simulink model "ThreePhaseVectorControl v2"  (R2020a)
settings: Solver=ode15s  StartTime=0.0  StopTime=2.5  MaxStep=1e-6  RelTol=1e-6
model workspace (MAT data in the model file):
  frequency = 1
values from neighbouring files (symbols this model uses):
  Buffer = 500    [PLLFYP.m]
  Ki_PLL = 0.005    [PLLFYP.m]
  Kp_PLL = 0.05    [PLLFYP.m]
  Kp_VSC = 500    [PLLFYP.m]
  Lf = 0.005    [PLLFYP.m]
  Lg = XR*Rg/(100*pi)    [PLLFYP.m]
  MPM_Ts = 1/5000    (= 0.0002)    [PLLFYP.m]
  Rf = 0.1    [PLLFYP.m]
  Rg = sqrt((1/(1+XR^2))*((500^2)/(Pn*SCR))^2)    [PLLFYP.m]
  Vdc = 2000    [PLLFYP.m]
  wL = 2*pi*50*Lf    (= 1.57079632679)    [PLLFYP.m]
  wn = 3000    [PLLFYP.m]
  zeta = 0.707    [PLLFYP.m]
undefined symbols (not defined in the file or in its folder): Ki_PQ, Kp_PQ, mpm_wc, plecs, Q, Q_KF, R, wb, wc, wc1, wc2
libraries: powerlib_meascontrol x57, powerlib x25, simulink x4, eeStairGenerator x4, powerlib_extras x2, cstblocks x2
(part 3 of 4)

== system ThreePhaseVectorControl v2/Vector Current Controller + PWM/KF_PLL/Kalman Filter-based PLL/Real Time Frequency Detection ==
  note: $x_{2_k}$
  note: $x_{1_k}$
  note: $\omega_k$
  r1 : Inport
  r2 : Inport  Port=2
  Trigger : TriggerPort  VariantControl=Variant  PortDimensions=1
  Add1 : Sum
  Discrete Derivative : simulink/Discrete/Discrete Derivative  gainval=1.0  ICPrevScaledInput=0.0  OutMin=[]  OutMax=[]  OutDataType=fixdt(1, 16)  OutScaling=2^-10  DoSatur=off
  Discrete Derivative1 : simulink/Discrete/Discrete Derivative  gainval=1.0  ICPrevScaledInput=0.0  OutMin=[]  OutMax=[]  OutDataType=fixdt(1, 16)  OutScaling=2^-10  DoSatur=off
  Divide4 : Product  Inputs=/*
  Product3 : Product
  Product4 : Product
  Square2 : Math  Operator=square  SaturateOnIntegerOverflow=on
  Square3 : Math  Operator=square  SaturateOnIntegerOverflow=on
  Subtract1 : Sum  Inputs=+-
  w_k : Outport
  wires:
  Subtract1/1 -> Divide4/2
  Product4/1 -> Subtract1/2
  r2/1 -> Square3/1, Discrete Derivative1/1, Product3/2
  Square3/1 -> Add1/2
  r1/1 -> Discrete Derivative/1, Product4/1, Square2/1
  Product3/1 -> Subtract1/1
  Square2/1 -> Add1/1
  Divide4/1 -> w_k/1
  Add1/1 -> Divide4/1
  Discrete Derivative1/1 -> Product4/2
  Discrete Derivative/1 -> Product3/1

== system ThreePhaseVectorControl v2/Vector Current Controller + PWM/KF_PLL/Kalman Filter-based PLL/abc-to-aphabetazero and Normalized ==
  note: $||v_{\alpha \beta k}^+||$
  note: $v_{\beta k}^+$
  note: $v_{\alpha k}^+$
  note: $r_{\beta_\omega}=cos(\theta_k^+)$
  note: $r_{\alpha__\omega}=sin(\theta_k^+)$
  note: $||v_{\alpha \beta k}^+||$
  Va S90 : Inport
  Vb S90 : Inport  Port=2
  Vc S90 : Inport  Port=3
  Trigger : TriggerPort  VariantControl=Variant  PortDimensions=1
  Add4 : Sum
  Demux : Demux  Outputs=3
  Divide : Product  Inputs=*/
  Divide2 : Product  Inputs=/*
  Mux : Mux  Inputs=3
  Square Root : Sqrt  SaturateOnIntegerOverflow=on
  Square6 : Math  Operator=square  SaturateOnIntegerOverflow=on
  Square7 : Math  Operator=square  SaturateOnIntegerOverflow=on
  Terminator : Terminator
  abc to Alpha-Beta-Zero : powerlib_meascontrol/Transformations/abc to Alpha-Beta-Zero
  r_bw : Outport
  r_aw : Outport  Port=2
  wires:
  abc to Alpha-Beta-Zero/1 -> Demux/1
  Square Root/1 -> Divide2/1, Divide/2
  Demux/2 -> Divide2/2, Square6/1
  Add4/1 -> Square Root/1
  Square7/1 -> Add4/1
  Square6/1 -> Add4/2
  Demux/1 -> Square7/1, Divide/1
  Demux/3 -> Terminator/1
  Mux/1 -> abc to Alpha-Beta-Zero/1
  Vc S90/1 -> Mux/3
  Divide2/1 -> r_bw/1
  Divide/1 -> r_aw/1
  Va S90/1 -> Mux/1
  Vb S90/1 -> Mux/2

== system ThreePhaseVectorControl v2/Vector Current Controller + PWM/KF_PLL/MPM (forcing Vq=0)/SRF-PLL for initialization ==
  VaB0 : Inport
  Add : Sum  Inputs=+-
  Add1 : Sum
  Alpha-Beta-Zero to dq0 : powerlib_meascontrol/Transformations/Alpha-Beta-Zero to dq0  Alignment=Aligned with phase A axis
  Constant : Constant  Value=2*pi
  Demux : Demux  Outputs=3
  Gain : Gain  Gain=Kp_PLL
  Integrator : Integrator  UpperSaturationLimit=2*pi  LowerSaturationLimit=0  IgnoreLimit=on
  Math Function : Math  Operator=mod  SignedPower=on  SaturateOnIntegerOverflow=on
  PI Controller : TransferFcn  Numerator=[1 Ki_PLL]  Denominator=[1 0]
  Terminator : Terminator
  Terminator1 : Terminator
  q reference : Step  Time=0  After=0  SampleTime=0
  w0 : Step  Time=0  After=2*pi*50  SampleTime=0
  SRF_theta : Outport
  wires:
  Demux/2 -> Add/1
  Math Function/1 -> SRF_theta/1, Alpha-Beta-Zero to dq0/2
  PI Controller/1 -> Add1/1
  q reference/1 -> Add/2
  Gain/1 -> PI Controller/1
  w0/1 -> Add1/2
  Demux/3 -> Terminator/1
  Add/1 -> Gain/1
  Alpha-Beta-Zero to dq0/1 -> Demux/1
  Constant/1 -> Math Function/2
  Integrator/1 -> Math Function/1
  Add1/1 -> Integrator/1
  VaB0/1 -> Alpha-Beta-Zero to dq0/1
  Demux/1 -> Terminator1/1

== system ThreePhaseVectorControl v2/Vector Current Controller + PWM/MPM/MPM (forcing Vq=0)/SRF-PLL for initialization ==
  VaB0 : Inport
  Add : Sum  Inputs=+-
  Add1 : Sum
  Alpha-Beta-Zero to dq0 : powerlib_meascontrol/Transformations/Alpha-Beta-Zero to dq0  Alignment=Aligned with phase A axis
  Constant : Constant  Value=2*pi
  Demux : Demux  Outputs=3
  Gain : Gain  Gain=Kp_PLL
  Integrator : Integrator  UpperSaturationLimit=2*pi  LowerSaturationLimit=0  IgnoreLimit=on
  Math Function : Math  Operator=mod  SignedPower=on  SaturateOnIntegerOverflow=on
  PI Controller : TransferFcn  Numerator=[1 Ki_PLL]  Denominator=[1 0]
  Terminator : Terminator
  Terminator1 : Terminator
  q reference : Step  Time=0  After=0  SampleTime=0
  w0 : Step  Time=0  After=2*pi*50  SampleTime=0
  SRF_theta : Outport
  wires:
  Demux/2 -> Add/1
  Math Function/1 -> SRF_theta/1, Alpha-Beta-Zero to dq0/2
  PI Controller/1 -> Add1/1
  q reference/1 -> Add/2
  Gain/1 -> PI Controller/1
  w0/1 -> Add1/2
  Demux/3 -> Terminator/1
  Add/1 -> Gain/1
  Alpha-Beta-Zero to dq0/1 -> Demux/1
  Constant/1 -> Math Function/2
  Integrator/1 -> Math Function/1
  Add1/1 -> Integrator/1
  VaB0/1 -> Alpha-Beta-Zero to dq0/1
  Demux/1 -> Terminator1/1

== system ThreePhaseVectorControl v2/Vector Current Controller + PWM/MPM/MPM (forcing Vq=0)/SRF-PLL for initialization1 ==
  VaB0 : Inport
  Add : Sum  Inputs=+-
  Add1 : Sum
  Alpha-Beta-Zero to dq0 : powerlib_meascontrol/Transformations/Alpha-Beta-Zero to dq0  Alignment=Aligned with phase A axis
  Constant : Constant  Value=2*pi
  Demux : Demux  Outputs=3
  Gain : Gain  Gain=Kp_PLL
  Integrator : Integrator  UpperSaturationLimit=2*pi  LowerSaturationLimit=0  IgnoreLimit=on
  Math Function : Math  Operator=mod  SignedPower=on  SaturateOnIntegerOverflow=on
  PI Controller : TransferFcn  Numerator=[1 Ki_PLL]  Denominator=[1 0]
  Terminator : Terminator
  Terminator1 : Terminator
  q reference : Step  Time=0  After=0  SampleTime=0
  w0 : Step  Time=0  After=2*pi*50  SampleTime=0
  SRF_theta : Outport
  wires:
  Demux/2 -> Add/1
  Math Function/1 -> SRF_theta/1, Alpha-Beta-Zero to dq0/2
  PI Controller/1 -> Add1/1
  q reference/1 -> Add/2
  Gain/1 -> PI Controller/1
  w0/1 -> Add1/2
  Demux/3 -> Terminator/1
  Add/1 -> Gain/1
  Alpha-Beta-Zero to dq0/1 -> Demux/1
  Constant/1 -> Math Function/2
  Integrator/1 -> Math Function/1
  Add1/1 -> Integrator/1
  VaB0/1 -> Alpha-Beta-Zero to dq0/1
  Demux/1 -> Terminator1/1

== system ThreePhaseVectorControl v2/Vector Current Controller + PWM/MPM/MPM (forcing Vq=0)/Vabc ==
  1 : Inport
  " InputMux " : Subsystem
      mask Display: disp('Mux')
  " S-Function " : S-Function  FunctionName=plecs  SFunctionDeploymentMode=off  EnableBusSupport=off
  wires:
  1/1 -> " InputMux "/1(In1)
  " InputMux "/1(Out) -> " S-Function "/1

== system ThreePhaseVectorControl v2/Vector Current Controller + PWM/MPM CF/MPM (forcing Vq=0)/SRF-PLL for initialization ==
  VaB0 : Inport
  Add : Sum  Inputs=+-
  Add1 : Sum
  Alpha-Beta-Zero to dq0 : powerlib_meascontrol/Transformations/Alpha-Beta-Zero to dq0  Alignment=Aligned with phase A axis
  Constant : Constant  Value=2*pi
  Demux : Demux  Outputs=3
  Gain : Gain  Gain=Kp_PLL
  Integrator : Integrator  UpperSaturationLimit=2*pi  LowerSaturationLimit=0  IgnoreLimit=on
  Math Function : Math  Operator=mod  SignedPower=on  SaturateOnIntegerOverflow=on
  PI Controller : TransferFcn  Numerator=[1 Ki_PLL]  Denominator=[1 0]
  Terminator : Terminator
  Terminator1 : Terminator
  q reference : Step  Time=0  After=0  SampleTime=0
  w0 : Step  Time=0  After=2*pi*50  SampleTime=0
  SRF_theta : Outport
  wires:
  Demux/2 -> Add/1
  Math Function/1 -> SRF_theta/1, Alpha-Beta-Zero to dq0/2
  PI Controller/1 -> Add1/1
  q reference/1 -> Add/2
  Gain/1 -> PI Controller/1
  w0/1 -> Add1/2
  Demux/3 -> Terminator/1
  Add/1 -> Gain/1
  Alpha-Beta-Zero to dq0/1 -> Demux/1
  Constant/1 -> Math Function/2
  Integrator/1 -> Math Function/1
  Add1/1 -> Integrator/1
  VaB0/1 -> Alpha-Beta-Zero to dq0/1
  Demux/1 -> Terminator1/1

== system ThreePhaseVectorControl v2/Vector Current Controller + PWM/MPM CF1/MPM (forcing Vq=0)/SRF-PLL for initialization ==
  VaB0 : Inport
  Add : Sum  Inputs=+-
  Add1 : Sum
  Alpha-Beta-Zero to dq0 : powerlib_meascontrol/Transformations/Alpha-Beta-Zero to dq0  Alignment=Aligned with phase A axis
  Constant : Constant  Value=2*pi
  Demux : Demux  Outputs=3
  Gain : Gain  Gain=Kp_PLL
  Integrator : Integrator  UpperSaturationLimit=2*pi  LowerSaturationLimit=0  IgnoreLimit=on
  Math Function : Math  Operator=mod  SignedPower=on  SaturateOnIntegerOverflow=on
  PI Controller : TransferFcn  Numerator=[1 Ki_PLL]  Denominator=[1 0]
  Terminator : Terminator
  Terminator1 : Terminator
  q reference : Step  Time=0  After=0  SampleTime=0
  w0 : Step  Time=0  After=2*pi*50  SampleTime=0
  SRF_theta : Outport
  wires:
  Demux/2 -> Add/1
  Math Function/1 -> SRF_theta/1, Alpha-Beta-Zero to dq0/2
  PI Controller/1 -> Add1/1
  q reference/1 -> Add/2
  Gain/1 -> PI Controller/1
  w0/1 -> Add1/2
  Demux/3 -> Terminator/1
  Add/1 -> Gain/1
  Alpha-Beta-Zero to dq0/1 -> Demux/1
  Constant/1 -> Math Function/2
  Integrator/1 -> Math Function/1
  Add1/1 -> Integrator/1
  VaB0/1 -> Alpha-Beta-Zero to dq0/1
  Demux/1 -> Terminator1/1

== system ThreePhaseVectorControl v2/Vector Current Controller + PWM/MPM//SRF CF/MPM (forcing Vq=0)/SRF-PLL for initialization ==
  VaB0 : Inport
  Add : Sum  Inputs=+-
  Add1 : Sum
  Alpha-Beta-Zero to dq0 : powerlib_meascontrol/Transformations/Alpha-Beta-Zero to dq0  Alignment=Aligned with phase A axis
  Constant : Constant  Value=2*pi
  Demux : Demux  Outputs=3
  Gain : Gain  Gain=Kp_PLL
  Integrator : Integrator  UpperSaturationLimit=2*pi  LowerSaturationLimit=0  IgnoreLimit=on
  Math Function : Math  Operator=mod  SignedPower=on  SaturateOnIntegerOverflow=on
  PI Controller : TransferFcn  Numerator=[1 Ki_PLL]  Denominator=[1 0]
  Terminator : Terminator
  Terminator1 : Terminator
  q reference : Step  Time=0  After=0  SampleTime=0
  w0 : Step  Time=0  After=2*pi*50  SampleTime=0
  SRF_theta : Outport
  wires:
  Demux/2 -> Add/1
  Math Function/1 -> SRF_theta/1, Alpha-Beta-Zero to dq0/2
  PI Controller/1 -> Add1/1
  q reference/1 -> Add/2
  Gain/1 -> PI Controller/1
  w0/1 -> Add1/2
  Demux/3 -> Terminator/1
  Add/1 -> Gain/1
  Alpha-Beta-Zero to dq0/1 -> Demux/1
  Constant/1 -> Math Function/2
  Integrator/1 -> Math Function/1
  Add1/1 -> Integrator/1
  VaB0/1 -> Alpha-Beta-Zero to dq0/1
  Demux/1 -> Terminator1/1

== system ThreePhaseVectorControl v2/Vector Current Controller + PWM/MPM//SRF CF/SRF_PLL/Vabc ==
  1 : Inport
  " InputMux " : Subsystem
      mask Display: disp('Mux')
  " S-Function " : S-Function  FunctionName=plecs  SFunctionDeploymentMode=off  EnableBusSupport=off
  wires:
  1/1 -> " InputMux "/1(In1)
  " InputMux "/1(Out) -> " S-Function "/1

== system ThreePhaseVectorControl v2/Vector Current Controller + PWM/MPM//SRF CF/SRF_PLL/Valphabeta ==
  1 : Inport
  " InputMux " : Subsystem
      mask Display: disp('Mux')
  " S-Function " : S-Function  FunctionName=plecs  SFunctionDeploymentMode=off  EnableBusSupport=off
  wires:
  1/1 -> " InputMux "/1(In1)
  " InputMux "/1(Out) -> " S-Function "/1

== system ThreePhaseVectorControl v2/Vector Current Controller + PWM/SRF_PLL/Vabc/ InputMux  ==
  In1 : Inport
  Convert1 : DataTypeConversion  SaturateOnIntegerOverflow=on  RndMeth=Zero
  Mux : Mux  Inputs=1
  Out : Outport
  wires:
  Convert1/1 -> Mux/1
  In1/1 -> Convert1/1
  Mux/1 -> Out/1

== system ThreePhaseVectorControl v2/Vector Current Controller + PWM/SRF_PLL/Valphabeta/ InputMux  ==
  In1 : Inport
  Convert1 : DataTypeConversion  SaturateOnIntegerOverflow=on  RndMeth=Zero
  Mux : Mux  Inputs=1
  Out : Outport
  wires:
  Convert1/1 -> Mux/1
  In1/1 -> Convert1/1
  Mux/1 -> Out/1

== system ThreePhaseVectorControl v2/Vector Current Controller + PWM/MPM/MPM (forcing Vq=0)/Vabc/ InputMux  ==
  In1 : Inport
  Convert1 : DataTypeConversion  SaturateOnIntegerOverflow=on  RndMeth=Zero
  Mux : Mux  Inputs=1
  Out : Outport
  wires:
  Convert1/1 -> Mux/1
  In1/1 -> Convert1/1
  Mux/1 -> Out/1

== system ThreePhaseVectorControl v2/Vector Current Controller + PWM/MPM//SRF CF/SRF_PLL/Vabc/ InputMux  ==
  In1 : Inport
  Convert1 : DataTypeConversion  SaturateOnIntegerOverflow=on  RndMeth=Zero
  Mux : Mux  Inputs=1
  Out : Outport
  wires:
  Convert1/1 -> Mux/1
  In1/1 -> Convert1/1
  Mux/1 -> Out/1

== system ThreePhaseVectorControl v2/Vector Current Controller + PWM/MPM//SRF CF/SRF_PLL/Valphabeta/ InputMux  ==
  In1 : Inport
  Convert1 : DataTypeConversion  SaturateOnIntegerOverflow=on  RndMeth=Zero
  Mux : Mux  Inputs=1
  Out : Outport
  wires:
  Convert1/1 -> Mux/1
  In1/1 -> Convert1/1
  Mux/1 -> Out/1

== matlab function ThreePhaseVectorControl v2/Vector Current Controller + PWM/MPM//SRF CF/MPM/MPM method 5 cycle ==
  data: x input; L input; timestep input; freq_guess input; outputfreq output
function outputfreq = Our_MPM_QR_pca(x,L,timestep,freq_guess)

%     Applies the Total Forward Backward Matrix Pencil Method to resolve the
%     synchrophasor of an input signal
%     Author: Lakshan Bernard, Sunny Goondram

% Inputs
% x:          one window of the timeseries
% L:          pencil parameter
% timestep:   time between sample points
% freq_guess: which phasors to report. NB: the method calculates all phasors
%             but the this just tells the algorithm to output phasor closest
%             to freq_guess
%             
% Outputs
% outputphasor:   a complex number representing the phasor relative to start
%                 of the window.
% outputfreq:     the frequency of the phasor. Note this is different to
%                 freq_guess
% eigS, residues: these contain all the frequency and phasor data

x = reshape(x, [], 1); %reshape data into column vector
N = length(x);
sampleoffset = (ceil(N/2)+1);
xold = x;

% Hyperparameters
DYNAMIC = 0;
if(DYNAMIC)
    epsilon=0.125;
    sys_order=floor((0.22/(50*timestep)));
else
    epsilon=0.05; %0.0050;
    sys_order=floor((N-sampleoffset)*1);
end

%% Filtering
    L1 = ceil(N/2);
    Y = hankel(x(1:N-L1), x(N-L1:N)); diagIdx = (N:-1:1)-L1;
    
    Y_mean = mean(Y,1);
    n = size(Y,1);
    matrix_mean = repmat(Y_mean,n,1); %creates a matrix with similar rows 
    centered_data = Y- matrix_mean;% centering the data by subtracting the mean
    M = ((centered_data')*centered_data)/(n-1);
    [V,D] = eig(M); %V are eigenvectors and D represents the eigenvalues 

    %sorting the eigen values in descending order
    lx = size(Y,2);
    eval = zeros(1,lx);
    eval = complex(eval, zeros(size(eval), class(eval)) );                      % Additional code added in
    for k = 1:lx
        eval(1,k) = D(k,k);
    end 
    [eval_sorted,I] = sort(eval,'descend');
    
    S = cumsum(abs(eval_sorted));
    limit = find((S/S(end))>0.9999999,1);
    if isempty(limit)                                                           % Additional code added in
        limit = 1;
    end
    limit = limit(1);
    evec_sorted = zeros(lx,limit);
    evec_sorted = complex(evec_sorted, zeros(size(evec_sorted), class(evec_sorted)) );    % Additional code added in
    for m =1:limit
        evec_sorted(:,m) = V(:,I(m));
    end
        
    %reconstruction
    princ_compon_limit = centered_data*evec_sorted;
    reconstructed = princ_compon_limit *(evec_sorted');
    reconstructed = reconstructed + matrix_mean;
    C = reconstructed;
 
    x1 = zeros(1,N);
    x1 = complex(x1, zeros(size(x1), class(x1)) );                              % Additional code added in
    for i=1:length(diagIdx) %averaging antidiagonals
        x1(i) = mean(diag(fliplr(C),diagIdx(i)));
    end    
    C = hankel(x1(1:N-L1), x1(N-L1:N)); 

    
%% Solving GEP

%perform the Column permutated QR decomposition for finding eigenvalues
%find the QR decomp for the all data matrix
[Q,R,E]=qr(C);

%rank estimation
order=0;

for i=1:length(diag(R))
    if abs(R(i,i))>=epsilon*abs(R(1,1))
        order=order+1;
    end
end

% Use permutation matrix to modify the Triangular R matrix
S=R*((E).');
% Create a new truncated pencil using the new matrix 
T1=S(1:order,1:L);
T2=S(1:order,2:L+1);
%modify the new pencil with diagonal of R matrix
Dinv=inv(diag(diag(R(1:order,1:order))));
T1dash=Dinv*T1;
T2dash=Dinv*T2;
%use the new pencil to find the eigenvalues
eigsS=eig(pinv(T2dash)*T1dash);
%remove the 0 eigenvalues;

eigsS(abs(eigsS)<10^-8)=[];
eigsS((abs(eigsS)<0.9)|(abs(eigsS)>1.1))=0;
order=length(eigsS);

%% Solving Complex Amplitudes
%form the linear system to solve for the complex amplitudes
ans_vec=xold(1+sampleoffset:sys_order+sampleoffset); %build answer vector (NB, this data hasnt been filtered :/)
coef_mat=zeros(sys_order,order);
coef_mat = complex(coef_mat, zeros(size(coef_mat), class(coef_mat)) );         % Additional code added in
for i=1:sys_order %build coefficient matrix
    for j=1:order
        coef_mat(i,j)=eigsS(j)^(i-1);
    end
end
residues=pinv(coef_mat)*ans_vec; %find the complex amplitudes


%% Estimating Frequency
freq = angle(eigsS)/(2*pi*timestep);
estfreq=freq_guess; %to report fundamental phasor replace with 50..
outputfreq = mean(freq( (freq>0.85*estfreq)&(freq<1.15*estfreq) ));

%% Reconstructing Phasor
%outputphasor = 2*sum(residues( (freq>0.85*freq_guess)&(freq<1.15*freq_guess) ));

== matlab function ThreePhaseVectorControl v2/Vector Current Controller + PWM/KF_PLL/KF//GAM/Kalman Filter/KF_Vb ==
  data: y_k input; v_fk output; R input; Q input; w_k input; V_fk_S90 output
function [v_fk, V_fk_S90] = fcn(y_k, R, Q, w_k)
 
persistent P_k;
persistent xhat_k;

% Initialize xhat and Phat
    if isempty(P_k)
        P_k = eye(2);
    end
    if isempty(xhat_k)
        xhat_k = zeros(2, 1);
    end
    
% Variables for KF
    Ts = 10e-6;       
    phi_k = [cos(w_k*Ts) sin(w_k*Ts); -sin(w_k*Ts) cos(w_k*Ts)];  
    F_k = [1 0];


K = phi_k * P_k * F_k' / (F_k * P_k * F_k' + R);        %K_gain * Phat_next * F_k' /(F_k*Phat_next*F_k' + R);    
xhat_k1 = phi_k * xhat_k + K * (y_k - F_k * xhat_k);
P_k1 = phi_k * P_k * phi_k' - K * F_k * P_k * phi_k' + Q;

xhat_k = xhat_k1;
P_k = P_k1;

% Output
v_fk = xhat_k1(1);
V_fk_S90 = xhat_k1(2);


 
end

== matlab function ThreePhaseVectorControl v2/Vector Current Controller + PWM/KF_PLL/KF//GAM/Kalman Filter/KF_Vc ==
  data: y_k input; v_fk output; R input; Q input; w_k input; V_fk_S90 output
function [v_fk, V_fk_S90] = fcn(y_k, R, Q, w_k)
 
persistent P_k;
persistent xhat_k;

% Initialize xhat and Phat
    if isempty(P_k)
        P_k = eye(2);
    end
    if isempty(xhat_k)
        xhat_k = zeros(2, 1);
    end

% Variables for KF
    Ts = 10e-6;       
    phi_k = [cos(w_k*Ts) sin(w_k*Ts); -sin(w_k*Ts) cos(w_k*Ts)];  %phi_k = [1 0; 0 1];
    F_k = [1 0];


K = phi_k * P_k * F_k' / (F_k * P_k * F_k' + R);        %K_gain * Phat_next * F_k' /(F_k*Phat_next*F_k' + R);    
xhat_k1 = phi_k * xhat_k + K * (y_k - F_k * xhat_k);
P_k1 = phi_k * P_k * phi_k' - K * F_k * P_k * phi_k' + Q;

xhat_k = xhat_k1;
P_k = P_k1;

% Output
v_fk = xhat_k1(1);
V_fk_S90 = xhat_k1(2);


 
end

== matlab function ThreePhaseVectorControl v2/Vector Current Controller + PWM/MPM CF1/MPM/MPM method 2 cycle ==
  data: x input; L input; timestep input; freq_guess input; outputfreq output
function outputfreq = Our_MPM_QR_pca(x,L,timestep,freq_guess)

%     Applies the Total Forward Backward Matrix Pencil Method to resolve the
%     synchrophasor of an input signal
%     Author: Lakshan Bernard, Sunny Goondram

% Inputs
% x:          one window of the timeseries
% L:          pencil parameter
% timestep:   time between sample points
% freq_guess: which phasors to report. NB: the method calculates all phasors
%             but the this just tells the algorithm to output phasor closest
%             to freq_guess
%             
% Outputs
% outputphasor:   a complex number representing the phasor relative to start
%                 of the window.
% outputfreq:     the frequency of the phasor. Note this is different to
%                 freq_guess
% eigS, residues: these contain all the frequency and phasor data

x = reshape(x, [], 1); %reshape data into column vector
N = length(x);
sampleoffset = (ceil(N/2)+1);
xold = x;

% Hyperparameters
DYNAMIC = 0;
if(DYNAMIC)
    epsilon=0.125;
    sys_order=floor((0.22/(50*timestep)));
else
    epsilon=0.005; %0.0050;
    sys_order=floor((N-sampleoffset)*1);
end

%% Filtering
    L1 = ceil(N/2);
    Y = hankel(x(1:N-L1), x(N-L1:N)); diagIdx = (N:-1:1)-L1;
    
    Y_mean = mean(Y,1);
    n = size(Y,1);
    matrix_mean = repmat(Y_mean,n,1); %creates a matrix with similar rows 
    centered_data = Y- matrix_mean;% centering the data by subtracting the mean
    M = ((centered_data')*centered_data)/(n-1);
    [V,D] = eig(M); %V are eigenvectors and D represents the eigenvalues 

    %sorting the eigen values in descending order
    lx = size(Y,2);
    eval = zeros(1,lx);
    eval = complex(eval, zeros(size(eval), class(eval)) );                      % Additional code added in
    for k = 1:lx
        eval(1,k) = D(k,k);
    end 
    [eval_sorted,I] = sort(eval,'descend');
    
    S = cumsum(abs(eval_sorted));
    limit = find((S/S(end))>0.9999999,1);
    if isempty(limit)                                                           % Additional code added in
        limit = 1;
    end
    limit = limit(1);
    evec_sorted = zeros(lx,limit);
    evec_sorted = complex(evec_sorted, zeros(size(evec_sorted), class(evec_sorted)) );    % Additional code added in
    for m =1:limit
        evec_sorted(:,m) = V(:,I(m));
    end
        
    %reconstruction
    princ_compon_limit = centered_data*evec_sorted;
    reconstructed = princ_compon_limit *(evec_sorted');
    reconstructed = reconstructed + matrix_mean;
    C = reconstructed;
 
    x1 = zeros(1,N);
    x1 = complex(x1, zeros(size(x1), class(x1)) );                              % Additional code added in
    for i=1:length(diagIdx) %averaging antidiagonals
        x1(i) = mean(diag(fliplr(C),diagIdx(i)));
    end    
    C = hankel(x1(1:N-L1), x1(N-L1:N)); 

    
%% Solving GEP

%perform the Column permutated QR decomposition for finding eigenvalues
%find the QR decomp for the all data matrix
[Q,R,E]=qr(C);

%rank estimation
order=0;

for i=1:length(diag(R))
    if abs(R(i,i))>=epsilon*abs(R(1,1))
        order=order+1;
    end
end

% Use permutation matrix to modify the Triangular R matrix
S=R*((E).');
% Create a new truncated pencil using the new matrix 
T1=S(1:order,1:L);
T2=S(1:order,2:L+1);
%modify the new pencil with diagonal of R matrix
Dinv=inv(diag(diag(R(1:order,1:order))));
T1dash=Dinv*T1;
T2dash=Dinv*T2;
%use the new pencil to find the eigenvalues
eigsS=eig(pinv(T2dash)*T1dash);
%remove the 0 eigenvalues;

eigsS(abs(eigsS)<10^-8)=[];
eigsS((abs(eigsS)<0.9)|(abs(eigsS)>1.1))=0;
order=length(eigsS);

%% Solving Complex Amplitudes
%form the linear system to solve for the complex amplitudes
ans_vec=xold(1+sampleoffset:sys_order+sampleoffset); %build answer vector (NB, this data hasnt been filtered :/)
coef_mat=zeros(sys_order,order);
coef_mat = complex(coef_mat, zeros(size(coef_mat), class(coef_mat)) );         % Additional code added in
for i=1:sys_order %build coefficient matrix
    for j=1:order
        coef_mat(i,j)=eigsS(j)^(i-1);
    end
end
residues=pinv(coef_mat)*ans_vec; %find the complex amplitudes


%% Estimating Frequency
freq = angle(eigsS)/(2*pi*timestep);
estfreq=freq_guess; %to report fundamental phasor replace with 50..
outputfreq = mean(freq( (freq>0.85*estfreq)&(freq<1.15*estfreq) ));

%% Reconstructing Phasor
%outputphasor = 2*sum(residues( (freq>0.85*freq_guess)&(freq<1.15*freq_guess) ));

== matlab function ThreePhaseVectorControl v2/Vector Current Controller + PWM/MPM CF1/MPM/MPM method 5 cycle ==
  data: x input; L input; timestep input; freq_guess input; outputfreq output
function outputfreq = Our_MPM_QR_pca(x,L,timestep,freq_guess)

%     Applies the Total Forward Backward Matrix Pencil Method to resolve the
%     synchrophasor of an input signal
%     Author: Lakshan Bernard, Sunny Goondram

% Inputs
% x:          one window of the timeseries
% L:          pencil parameter
% timestep:   time between sample points
% freq_guess: which phasors to report. NB: the method calculates all phasors
%             but the this just tells the algorithm to output phasor closest
%             to freq_guess
%             
% Outputs
% outputphasor:   a complex number representing the phasor relative to start
%                 of the window.
% outputfreq:     the frequency of the phasor. Note this is different to
%                 freq_guess
% eigS, residues: these contain all the frequency and phasor data

x = reshape(x, [], 1); %reshape data into column vector
N = length(x);
sampleoffset = (ceil(N/2)+1);
xold = x;

% Hyperparameters
DYNAMIC = 0;
if(DYNAMIC)
    epsilon=0.125;
    sys_order=floor((0.22/(50*timestep)));
else
    epsilon=0.05; %0.0050;
    sys_order=floor((N-sampleoffset)*1);
end

%% Filtering
    L1 = ceil(N/2);
    Y = hankel(x(1:N-L1), x(N-L1:N)); diagIdx = (N:-1:1)-L1;
    
    Y_mean = mean(Y,1);
    n = size(Y,1);
    matrix_mean = repmat(Y_mean,n,1); %creates a matrix with similar rows 
    centered_data = Y- matrix_mean;% centering the data by subtracting the mean
    M = ((centered_data')*centered_data)/(n-1);
    [V,D] = eig(M); %V are eigenvectors and D represents the eigenvalues 

    %sorting the eigen values in descending order
    lx = size(Y,2);
    eval = zeros(1,lx);
    eval = complex(eval, zeros(size(eval), class(eval)) );                      % Additional code added in
    for k = 1:lx
        eval(1,k) = D(k,k);
    end 
    [eval_sorted,I] = sort(eval,'descend');
    
    S = cumsum(abs(eval_sorted));
    limit = find((S/S(end))>0.9999999,1);
    if isempty(limit)                                                           % Additional code added in
        limit = 1;
    end
    limit = limit(1);
    evec_sorted = zeros(lx,limit);
    evec_sorted = complex(evec_sorted, zeros(size(evec_sorted), class(evec_sorted)) );    % Additional code added in
    for m =1:limit
        evec_sorted(:,m) = V(:,I(m));
    end
        
    %reconstruction
    princ_compon_limit = centered_data*evec_sorted;
    reconstructed = princ_compon_limit *(evec_sorted');
    reconstructed = reconstructed + matrix_mean;
    C = reconstructed;
 
    x1 = zeros(1,N);
    x1 = complex(x1, zeros(size(x1), class(x1)) );                              % Additional code added in
    for i=1:length(diagIdx) %averaging antidiagonals
        x1(i) = mean(diag(fliplr(C),diagIdx(i)));
    end    
    C = hankel(x1(1:N-L1), x1(N-L1:N)); 

    
%% Solving GEP

%perform the Column permutated QR decomposition for finding eigenvalues
%find the QR decomp for the all data matrix
[Q,R,E]=qr(C);

%rank estimation
order=0;

for i=1:length(diag(R))
    if abs(R(i,i))>=epsilon*abs(R(1,1))
        order=order+1;
    end
end

% Use permutation matrix to modify the Triangular R matrix
S=R*((E).');
% Create a new truncated pencil using the new matrix 
T1=S(1:order,1:L);
T2=S(1:order,2:L+1);
%modify the new pencil with diagonal of R matrix
Dinv=inv(diag(diag(R(1:order,1:order))));
T1dash=Dinv*T1;
T2dash=Dinv*T2;
%use the new pencil to find the eigenvalues
eigsS=eig(pinv(T2dash)*T1dash);
%remove the 0 eigenvalues;

eigsS(abs(eigsS)<10^-8)=[];
eigsS((abs(eigsS)<0.9)|(abs(eigsS)>1.1))=0;
order=length(eigsS);

%% Solving Complex Amplitudes
%form the linear system to solve for the complex amplitudes
ans_vec=xold(1+sampleoffset:sys_order+sampleoffset); %build answer vector (NB, this data hasnt been filtered :/)
coef_mat=zeros(sys_order,order);
coef_mat = complex(coef_mat, zeros(size(coef_mat), class(coef_mat)) );         % Additional code added in
for i=1:sys_order %build coefficient matrix
    for j=1:order
        coef_mat(i,j)=eigsS(j)^(i-1);
    end
end
residues=pinv(coef_mat)*ans_vec; %find the complex amplitudes


%% Estimating Frequency
freq = angle(eigsS)/(2*pi*timestep);
estfreq=freq_guess; %to report fundamental phasor replace with 50..
outputfreq = mean(freq( (freq>0.85*estfreq)&(freq<1.15*estfreq) ));

%% Reconstructing Phasor
%outputphasor = 2*sum(residues( (freq>0.85*freq_guess)&(freq<1.15*freq_guess) ));

== matlab function ThreePhaseVectorControl v2/Vector Current Controller + PWM/MPM/MPM/MPM method ==
  data: x input; L input; timestep input; freq_guess input; outputfreq output
function outputfreq = Our_MPM_QR_pca(x,L,timestep,freq_guess)

%     Applies the Total Forward Backward Matrix Pencil Method to resolve the
%     synchrophasor of an input signal
%     Author: Lakshan Bernard, Sunny Goondram

% Inputs
% x:          one window of the timeseries
% L:          pencil parameter
% timestep:   time between sample points
% freq_guess: which phasors to report. NB: the method calculates all phasors
%             but the this just tells the algorithm to output phasor closest
%             to freq_guess
%             
% Outputs
% outputphasor:   a complex number representing the phasor relative to start
%                 of the window.
% outputfreq:     the frequency of the phasor. Note this is different to
%                 freq_guess
% eigS, residues: these contain all the frequency and phasor data

x = reshape(x, [], 1); %reshape data into column vector
N = length(x);
sampleoffset = (ceil(N/2)+1);
xold = x;

persistent f0;
if isempty(f0)
    f0 = freq_guess;
end

% Hyperparameters
DYNAMIC = 0;
if(DYNAMIC)
    epsilon=0.125;
    sys_order=floor((0.22/(50*timestep)));
else
    epsilon= 0.15;  %0.0050;
    sys_order=floor((N-sampleoffset)*1);
end

%% Filtering
    L1 = ceil(N/2);
    Y = hankel(x(1:N-L1), x(N-L1:N)); diagIdx = (N:-1:1)-L1;
    
    Y_mean = mean(Y,1);
    n = size(Y,1);
    matrix_mean = repmat(Y_mean,n,1); %creates a matrix with similar rows 
    centered_data = Y- matrix_mean;% centering the data by subtracting the mean
    M = ((centered_data')*centered_data)/(n-1);
    [V,D] = eig(M); %V are eigenvectors and D represents the eigenvalues 

    %sorting the eigen values in descending order
    lx = size(Y,2);
    eval = zeros(1,lx);
    eval = complex(eval, zeros(size(eval), class(eval)) );                      % Additional code added in
    for k = 1:lx
        eval(1,k) = D(k,k);
    end 
    [eval_sorted,I] = sort(eval,'descend');
    
    S = cumsum(abs(eval_sorted));
    limit = find((S/S(end))>0.9999999,1);
    if isempty(limit)                                                           % Additional code added in
        limit = 1;
    end
    limit = limit(1);
    evec_sorted = zeros(lx,limit);
    evec_sorted = complex(evec_sorted, zeros(size(evec_sorted), class(evec_sorted)) );    % Additional code added in
    for m =1:limit
        evec_sorted(:,m) = V(:,I(m));
    end
        
    %reconstruction
    princ_compon_limit = centered_data*evec_sorted;
    reconstructed = princ_compon_limit *(evec_sorted');
    reconstructed = reconstructed + matrix_mean;
    C = reconstructed;
 
    x1 = zeros(1,N);
    x1 = complex(x1, zeros(size(x1), class(x1)) );                              % Additional code added in
    for i=1:length(diagIdx) %averaging antidiagonals
        x1(i) = mean(diag(fliplr(C),diagIdx(i)));
    end    
    C = hankel(x1(1:N-L1), x1(N-L1:N)); 

    
%% Solving GEP

%perform the Column permutated QR decomposition for finding eigenvalues
%find the QR decomp for the all data matrix
[Q,R,E]=qr(C);

%rank estimation
order=0;

for i=1:length(diag(R))
    if abs(R(i,i))>=epsilon*abs(R(1,1))
        order=order+1;
    end
end

% Use permutation matrix to modify the Triangular R matrix
S=R*((E).');
% Create a new truncated pencil using the new matrix 
T1=S(1:order,1:L);
T2=S(1:order,2:L+1);
%modify the new pencil with diagonal of R matrix
Dinv=inv(diag(diag(R(1:order,1:order))));
T1dash=Dinv*T1;
T2dash=Dinv*T2;
%use the new pencil to find the eigenvalues
eigsS=eig(pinv(T2dash)*T1dash);
%remove the 0 eigenvalues;

eigsS(abs(eigsS)<10^-8)=[];
eigsS((abs(eigsS)<0.9)|(abs(eigsS)>1.1))=0;
order=length(eigsS);

%% Solving Complex Amplitudes
%form the linear system to solve for the complex amplitudes
ans_vec=xold(1+sampleoffset:sys_order+sampleoffset); %build answer vector (NB, this data hasnt been filtered :/)
coef_mat=zeros(sys_order,order);
coef_mat = complex(coef_mat, zeros(size(coef_mat), class(coef_mat)) );         % Additional code added in
for i=1:sys_order %build coefficient matrix
    for j=1:order
        coef_mat(i,j)=eigsS(j)^(i-1);
    end
end
residues=pinv(coef_mat)*ans_vec; %find the complex amplitudes


%% Estimating Frequency
freq = angle(eigsS)/(2*pi*timestep);
estfreq=freq_guess; %to report fundamental phasor replace with 50..
outputfreq_temp = mean(freq( (freq>0.85*estfreq)&(freq<1.15*estfreq) )); %mean(freq( (freq>0.85*estfreq)&(freq<1.15*estfreq) ));
 
if (outputfreq_temp < 1000)&&(outputfreq_temp > 0)
     f0 = outputfreq_temp;
else
     outputfreq_temp = f0;
end

outputfreq = outputfreq_temp;
 

%% Reconstructing Phasor
% outputphasor = 2*sum(residues( (freq>0.9*freq_guess)&(freq<1.1*freq_guess) ));
% 
% outputphase = angle(outputphasor);

== matlab function ThreePhaseVectorControl v2/Vector Current Controller + PWM/CF 2/MPM/MPM method ==
  data: x input; L input; timestep input; freq_guess input; outputfreq output
function outputfreq = Our_MPM_QR_pca(x,L,timestep,freq_guess)

%     Applies the Total Forward Backward Matrix Pencil Method to resolve the
%     synchrophasor of an input signal
%     Author: Lakshan Bernard, Sunny Goondram

% Inputs
% x:          one window of the timeseries
% L:          pencil parameter
% timestep:   time between sample points
% freq_guess: which phasors to report. NB: the method calculates all phasors
%             but the this just tells the algorithm to output phasor closest
%             to freq_guess
%             
% Outputs
% outputphasor:   a complex number representing the phasor relative to start
%                 of the window.
% outputfreq:     the frequency of the phasor. Note this is different to
%                 freq_guess
% eigS, residues: these contain all the frequency and phasor data

x = reshape(x, [], 1); %reshape data into column vector
N = length(x);
sampleoffset = (ceil(N/2)+1);
xold = x;

persistent f0;
if isempty(f0)
    f0 = freq_guess;
end

% Hyperparameters
DYNAMIC = 0;
if(DYNAMIC)
    epsilon=0.125;
    sys_order=floor((0.22/(50*timestep)));
else
    epsilon= 0.725;  %0.0050;
    sys_order=floor((N-sampleoffset)*1);
end

%% Filtering
    L1 = ceil(N/2);
    Y = hankel(x(1:N-L1), x(N-L1:N)); diagIdx = (N:-1:1)-L1;
    
    Y_mean = mean(Y,1);
    n = size(Y,1);
    matrix_mean = repmat(Y_mean,n,1); %creates a matrix with similar rows 
    centered_data = Y- matrix_mean;% centering the data by subtracting the mean
    M = ((centered_data')*centered_data)/(n-1);
    [V,D] = eig(M); %V are eigenvectors and D represents the eigenvalues 

    %sorting the eigen values in descending order
    lx = size(Y,2);
    eval = zeros(1,lx);
    eval = complex(eval, zeros(size(eval), class(eval)) );                      % Additional code added in
    for k = 1:lx
        eval(1,k) = D(k,k);
    end 
    [eval_sorted,I] = sort(eval,'descend');
    
    S = cumsum(abs(eval_sorted));
    limit = find((S/S(end))>0.9999999,1);
    if isempty(limit)                                                           % Additional code added in
        limit = 1;
    end
    limit = limit(1);
    evec_sorted = zeros(lx,limit);
    evec_sorted = complex(evec_sorted, zeros(size(evec_sorted), class(evec_sorted)) );    % Additional code added in
    for m =1:limit
        evec_sorted(:,m) = V(:,I(m));
    end
        
    %reconstruction
    princ_compon_limit = centered_data*evec_sorted;
    reconstructed = princ_compon_limit *(evec_sorted');
    reconstructed = reconstructed + matrix_mean;
    C = reconstructed;
 
    x1 = zeros(1,N);
    x1 = complex(x1, zeros(size(x1), class(x1)) );                              % Additional code added in
    for i=1:length(diagIdx) %averaging antidiagonals
        x1(i) = mean(diag(fliplr(C),diagIdx(i)));
    end    
    C = hankel(x1(1:N-L1), x1(N-L1:N)); 

    
%% Solving GEP

%perform the Column permutated QR decomposition for finding eigenvalues
%find the QR decomp for the all data matrix
[Q,R,E]=qr(C);

%rank estimation
order=0;

for i=1:length(diag(R))
    if abs(R(i,i))>=epsilon*abs(R(1,1))
        order=order+1;
    end
end

% Use permutation matrix to modify the Triangular R matrix
S=R*((E).');
% Create a new truncated pencil using the new matrix 
T1=S(1:order,1:L);
T2=S(1:order,2:L+1);
%modify the new pencil with diagonal of R matrix
Dinv=inv(diag(diag(R(1:order,1:order))));
T1dash=Dinv*T1;
T2dash=Dinv*T2;
%use the new pencil to find the eigenvalues
eigsS=eig(pinv(T2dash)*T1dash);
%remove the 0 eigenvalues;

eigsS(abs(eigsS)<10^-8)=[];
eigsS((abs(eigsS)<0.9)|(abs(eigsS)>1.1))=0;
order=length(eigsS);

%% Solving Complex Amplitudes
%form the linear system to solve for the complex amplitudes
ans_vec=xold(1+sampleoffset:sys_order+sampleoffset); %build answer vector (NB, this data hasnt been filtered :/)
coef_mat=zeros(sys_order,order);
coef_mat = complex(coef_mat, zeros(size(coef_mat), class(coef_mat)) );         % Additional code added in
for i=1:sys_order %build coefficient matrix
    for j=1:order
        coef_mat(i,j)=eigsS(j)^(i-1);
    end
end
residues=pinv(coef_mat)*ans_vec; %find the complex amplitudes


%% Estimating Frequency
freq = angle(eigsS)/(2*pi*timestep);
estfreq=freq_guess; %to report fundamental phasor replace with 50..
outputfreq_temp = mean(freq( (freq>0.2*estfreq)&(freq<2.0*estfreq) )); %mean(freq( (freq>0.85*estfreq)&(freq<1.15*estfreq) ));

if (outputfreq_temp < 1000)&&(outputfreq_temp > 0)
    f0 = outputfreq_temp;
else
    outputfreq_temp = f0;
end
 
 outputfreq = outputfreq_temp;

%% Reconstructing Phasor
%outputphasor = 2*sum(residues( (freq>0.85*freq_guess)&(freq<1.15*freq_guess) ));

== matlab function ThreePhaseVectorControl v2/Vector Current Controller + PWM/CF 2/MATLAB Function ==
  data: G1 output; ROCOF input; G2 output
function [G1, G2] = fcn(ROCOF)

min_threshold = 1800;
max_threshold = 3500;

if (ROCOF < min_threshold)  % Steady state
    G1 = 0;
elseif (min_threshold <= ROCOF)&&(ROCOF < max_threshold)
    G1 = (ROCOF - min_threshold)/(max_threshold - min_threshold);
else 
    G1 = 1;
end

G2 = 1 - G1; % MPM weight

end

== matlab function ThreePhaseVectorControl v2/Vector Current Controller + PWM/CF/MPM/MPM method ==
  data: x input; L input; timestep input; freq_guess input; outputfreq output
function outputfreq = Our_MPM_QR_pca(x,L,timestep,freq_guess)

%     Applies the Total Forward Backward Matrix Pencil Method to resolve the
%     synchrophasor of an input signal
%     Author: Lakshan Bernard, Sunny Goondram

% Inputs
% x:          one window of the timeseries
% L:          pencil parameter
% timestep:   time between sample points
% freq_guess: which phasors to report. NB: the method calculates all phasors
%             but the this just tells the algorithm to output phasor closest
%             to freq_guess
%             
% Outputs
% outputphasor:   a complex number representing the phasor relative to start
%                 of the window.
% outputfreq:     the frequency of the phasor. Note this is different to
%                 freq_guess
% eigS, residues: these contain all the frequency and phasor data

x = reshape(x, [], 1); %reshape data into column vector
N = length(x);
sampleoffset = (ceil(N/2)+1);
xold = x;

persistent f0;
if isempty(f0)
    f0 = freq_guess;
end

% Hyperparameters
DYNAMIC = 0;
if(DYNAMIC)
    epsilon=0.125;
    sys_order=floor((0.22/(50*timestep)));
else
    epsilon= 0.95;  %0.0050;
    sys_order=floor((N-sampleoffset)*1);
end

%% Filtering
    L1 = ceil(N/2);
    Y = hankel(x(1:N-L1), x(N-L1:N)); diagIdx = (N:-1:1)-L1;
    
    Y_mean = mean(Y,1);
    n = size(Y,1);
    matrix_mean = repmat(Y_mean,n,1); %creates a matrix with similar rows 
    centered_data = Y- matrix_mean;% centering the data by subtracting the mean
    M = ((centered_data')*centered_data)/(n-1);
    [V,D] = eig(M); %V are eigenvectors and D represents the eigenvalues 

    %sorting the eigen values in descending order
    lx = size(Y,2);
    eval = zeros(1,lx);
    eval = complex(eval, zeros(size(eval), class(eval)) );                      % Additional code added in
    for k = 1:lx
        eval(1,k) = D(k,k);
    end 
    [eval_sorted,I] = sort(eval,'descend');
    
    S = cumsum(abs(eval_sorted));
    limit = find((S/S(end))>0.9999999,1);
    if isempty(limit)                                                           % Additional code added in
        limit = 1;
    end
    limit = limit(1);
    evec_sorted = zeros(lx,limit);
    evec_sorted = complex(evec_sorted, zeros(size(evec_sorted), class(evec_sorted)) );    % Additional code added in
    for m =1:limit
        evec_sorted(:,m) = V(:,I(m));
    end
        
    %reconstruction
    princ_compon_limit = centered_data*evec_sorted;
    reconstructed = princ_compon_limit *(evec_sorted');
    reconstructed = reconstructed + matrix_mean;
    C = reconstructed;
 
    x1 = zeros(1,N);
    x1 = complex(x1, zeros(size(x1), class(x1)) );                              % Additional code added in
    for i=1:length(diagIdx) %averaging antidiagonals
        x1(i) = mean(diag(fliplr(C),diagIdx(i)));
    end    
    C = hankel(x1(1:N-L1), x1(N-L1:N)); 

    
%% Solving GEP

%perform the Column permutated QR decomposition for finding eigenvalues
%find the QR decomp for the all data matrix
[Q,R,E]=qr(C);

%rank estimation
order=0;

for i=1:length(diag(R))
    if abs(R(i,i))>=epsilon*abs(R(1,1))
        order=order+1;
    end
end

% Use permutation matrix to modify the Triangular R matrix
S=R*((E).');
% Create a new truncated pencil using the new matrix 
T1=S(1:order,1:L);
T2=S(1:order,2:L+1);
%modify the new pencil with diagonal of R matrix
Dinv=inv(diag(diag(R(1:order,1:order))));
T1dash=Dinv*T1;
T2dash=Dinv*T2;
%use the new pencil to find the eigenvalues
eigsS=eig(pinv(T2dash)*T1dash);
%remove the 0 eigenvalues;

eigsS(abs(eigsS)<10^-8)=[];
eigsS((abs(eigsS)<0.9)|(abs(eigsS)>1.1))=0;
order=length(eigsS);

%% Solving Complex Amplitudes
%form the linear system to solve for the complex amplitudes
ans_vec=xold(1+sampleoffset:sys_order+sampleoffset); %build answer vector (NB, this data hasnt been filtered :/)
coef_mat=zeros(sys_order,order);
coef_mat = complex(coef_mat, zeros(size(coef_mat), class(coef_mat)) );         % Additional code added in
for i=1:sys_order %build coefficient matrix
    for j=1:order
        coef_mat(i,j)=eigsS(j)^(i-1);
    end
end
residues=pinv(coef_mat)*ans_vec; %find the complex amplitudes


%% Estimating Frequency
freq = angle(eigsS)/(2*pi*timestep);
estfreq=freq_guess; %to report fundamental phasor replace with 50..
outputfreq_temp = mean(freq( (freq>0.95*estfreq)&(freq<1.05*estfreq) )); %mean(freq( (freq>0.85*estfreq)&(freq<1.15*estfreq) ));

if (outputfreq_temp < 100)&&(outputfreq_temp > 0)
    f0 = outputfreq_temp;
else
    outputfreq_temp = f0;
end
 
 outputfreq = outputfreq_temp;

%% Reconstructing Phasor
%outputphasor = 2*sum(residues( (freq>0.85*freq_guess)&(freq<1.15*freq_guess) ));

== matlab function ThreePhaseVectorControl v2/Vector Current Controller + PWM/CF (2)/MATLAB Function ==
  settings: updateMethod=DISCRETE
  data: wc output; ROCOF input; clk input
function wc  = fcn(ROCOF, clk)

persistent time; persistent trig; persistent prev_wc;

if isempty(time)
    time = 0;
end
if isempty(trig)
    trig = 0;
end
if isempty(prev_wc)
    prev_wc = 2*pi*783445;
end

threshold = 4000;

if (ROCOF >= threshold)  % Dynamic
    wc = 2*pi*5;       
else                     % Steady state
    wc = 2*pi*783445;   
end

if (prev_wc < wc)&&(trig == 0)
    time = clk;
    wc = 2*pi*5;
    trig = 1;
elseif (prev_wc < wc)&&(clk < time + 0.1)&&(trig == 1)
    wc = 2*pi*5;
elseif (prev_wc < wc)&&(clk == time + 0.1)&&(trig == 1)
    wc = 2*pi*783445;
    trig = 0;
elseif (prev_wc == wc)&&(trig == 1)
    time = clk;
end

prev_wc = wc;

end

== matlab function ThreePhaseVectorControl v2/Vector Current Controller + PWM/CF (2)/MPM/MPM method ==
  data: x input; L input; timestep input; freq_guess input; outputfreq output
function outputfreq = Our_MPM_QR_pca(x,L,timestep,freq_guess)

%     Applies the Total Forward Backward Matrix Pencil Method to resolve the
%     synchrophasor of an input signal
%     Author: Lakshan Bernard, Sunny Goondram

% Inputs
% x:          one window of the timeseries
% L:          pencil parameter
% timestep:   time between sample points
% freq_guess: which phasors to report. NB: the method calculates all phasors
%             but the this just tells the algorithm to output phasor closest
%             to freq_guess
%             
% Outputs
% outputphasor:   a complex number representing the phasor relative to start
%                 of the window.
% outputfreq:     the frequency of the phasor. Note this is different to
%                 freq_guess
% eigS, residues: these contain all the frequency and phasor data

x = reshape(x, [], 1); %reshape data into column vector
N = length(x);
sampleoffset = (ceil(N/2)+1);
xold = x;

persistent f0;
if isempty(f0)
    f0 = freq_guess;
end

% Hyperparameters
DYNAMIC = 0;
if(DYNAMIC)
    epsilon=0.125;
    sys_order=floor((0.22/(50*timestep)));
else
    epsilon= 0.725;  %0.0050;
    sys_order=floor((N-sampleoffset)*1);
end

%% Filtering
    L1 = ceil(N/2);
    Y = hankel(x(1:N-L1), x(N-L1:N)); diagIdx = (N:-1:1)-L1;
    
    Y_mean = mean(Y,1);
    n = size(Y,1);
    matrix_mean = repmat(Y_mean,n,1); %creates a matrix with similar rows 
    centered_data = Y- matrix_mean;% centering the data by subtracting the mean
    M = ((centered_data')*centered_data)/(n-1);
    [V,D] = eig(M); %V are eigenvectors and D represents the eigenvalues 

    %sorting the eigen values in descending order
    lx = size(Y,2);
    eval = zeros(1,lx);
    eval = complex(eval, zeros(size(eval), class(eval)) );                      % Additional code added in
    for k = 1:lx
        eval(1,k) = D(k,k);
    end 
    [eval_sorted,I] = sort(eval,'descend');
    
    S = cumsum(abs(eval_sorted));
    limit = find((S/S(end))>0.9999999,1);
    if isempty(limit)                                                           % Additional code added in
        limit = 1;
    end
    limit = limit(1);
    evec_sorted = zeros(lx,limit);
    evec_sorted = complex(evec_sorted, zeros(size(evec_sorted), class(evec_sorted)) );    % Additional code added in
    for m =1:limit
        evec_sorted(:,m) = V(:,I(m));
    end
        
    %reconstruction
    princ_compon_limit = centered_data*evec_sorted;
    reconstructed = princ_compon_limit *(evec_sorted');
    reconstructed = reconstructed + matrix_mean;
    C = reconstructed;
 
    x1 = zeros(1,N);
    x1 = complex(x1, zeros(size(x1), class(x1)) );                              % Additional code added in
    for i=1:length(diagIdx) %averaging antidiagonals
        x1(i) = mean(diag(fliplr(C),diagIdx(i)));
    end    
    C = hankel(x1(1:N-L1), x1(N-L1:N)); 

    
%% Solving GEP

%perform the Column permutated QR decomposition for finding eigenvalues
%find the QR decomp for the all data matrix
[Q,R,E]=qr(C);

%rank estimation
order=0;

for i=1:length(diag(R))
    if abs(R(i,i))>=epsilon*abs(R(1,1))
        order=order+1;
    end
end

% Use permutation matrix to modify the Triangular R matrix
S=R*((E).');
% Create a new truncated pencil using the new matrix 
T1=S(1:order,1:L);
T2=S(1:order,2:L+1);
%modify the new pencil with diagonal of R matrix
Dinv=inv(diag(diag(R(1:order,1:order))));
T1dash=Dinv*T1;
T2dash=Dinv*T2;
%use the new pencil to find the eigenvalues
eigsS=eig(pinv(T2dash)*T1dash);
%remove the 0 eigenvalues;

eigsS(abs(eigsS)<10^-8)=[];
eigsS((abs(eigsS)<0.9)|(abs(eigsS)>1.1))=0;
order=length(eigsS);

%% Solving Complex Amplitudes
%form the linear system to solve for the complex amplitudes
ans_vec=xold(1+sampleoffset:sys_order+sampleoffset); %build answer vector (NB, this data hasnt been filtered :/)
coef_mat=zeros(sys_order,order);
coef_mat = complex(coef_mat, zeros(size(coef_mat), class(coef_mat)) );         % Additional code added in
for i=1:sys_order %build coefficient matrix
    for j=1:order
        coef_mat(i,j)=eigsS(j)^(i-1);
    end
end
residues=pinv(coef_mat)*ans_vec; %find the complex amplitudes


%% Estimating Frequency
freq = angle(eigsS)/(2*pi*timestep);
estfreq=freq_guess; %to report fundamental phasor replace with 50..
outputfreq_temp = mean(freq( (freq>0.85*estfreq)&(freq<1.15*estfreq) )); 

if (outputfreq_temp < 1000)&&(outputfreq_temp > 0)
    f0 = outputfreq_temp;
else
    outputfreq_temp = f0;
end
 
 outputfreq = outputfreq_temp;

%% Reconstructing Phasor
%outputphasor = 2*sum(residues( (freq>0.85*freq_guess)&(freq<1.15*freq_guess) ));
